simulink library "require"  (Simulink 8.1)
settings: Solver=ode45  StartTime=0.0  StopTime=10.0  RelTol=1e-3
settings Model: Creator=aeagr  LastModifiedBy=dejanira

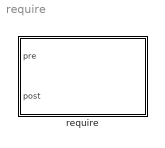
== system require ==
  require : Subsystem  TreatAsAtomicUnit=on  mask(Require){dummy=0}
      mask prompts: dummy "Random"
      mask Display:
      | image('assert.jpg')
      | port_label('input',1,'pre')
      | port_label('input',2,'post')

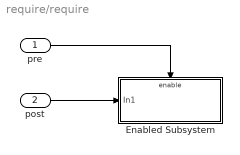
== system require/require ==
  pre : Inport
  post : Inport  Port=2
  Enabled Subsystem : Subsystem  TreatAsAtomicUnit=on
  wires:
  post/1 -> Enabled Subsystem/1(In1)
  pre/1 -> Enabled Subsystem/Enable

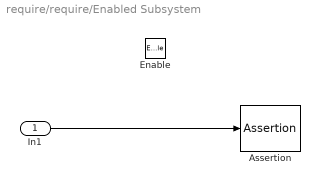
== system require/require/Enabled Subsystem ==
  In1 : Inport
  Enable : EnablePort
  Assertion : Assertion  StopWhenAssertionFail=off
  wires:
  In1/1 -> Assertion/1
